simulink model "sampleModel52"  (R2021b)
settings: Solver=VariableStepAuto  StartTime=0.0  StopTime=10.0  RelTol=1e-3
undefined symbols (not defined in the file or in its folder): magnitude
libraries: simulink x3
settings Model: Creator=user  LastModifiedBy=user

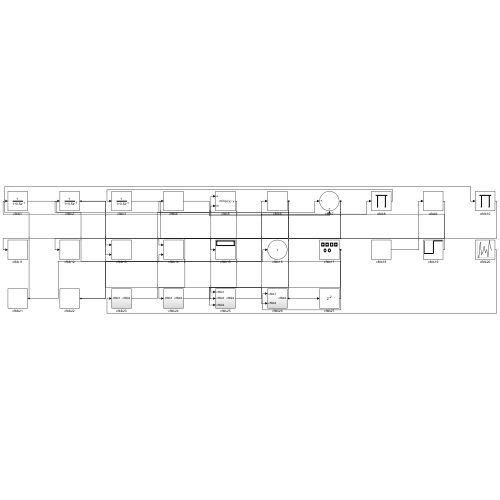
[thumbnail: Simulink's stored preview of the top-level diagram]
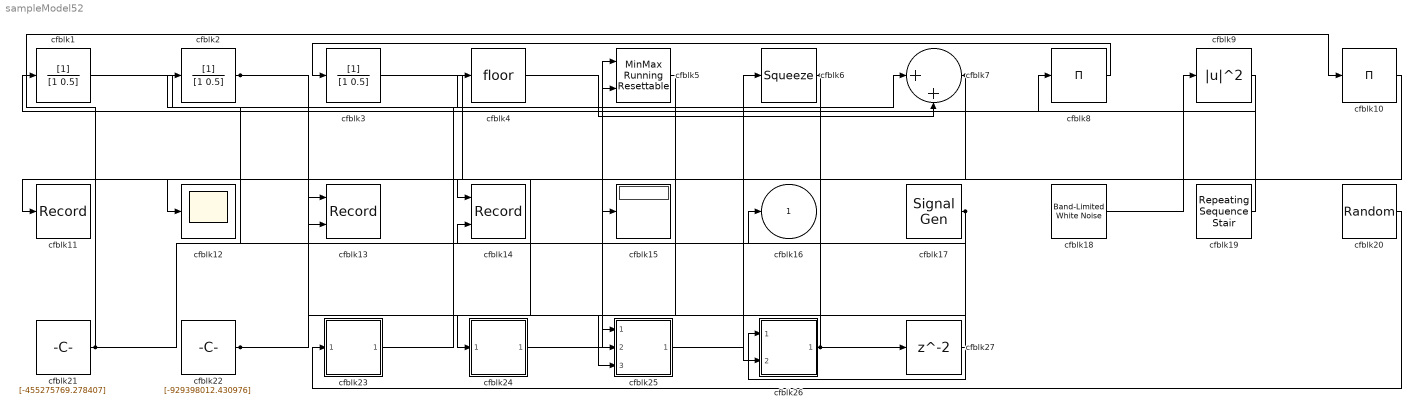
== system sampleModel52 ==
  cfblk1 : DiscreteFilter  SampleTime=1
  cfblk10 : Product  Inputs=*
  cfblk11 : Record  FileSettingsInternal="{\"entries\":[{\"content\":{\"excelSettings\":{\"content\":{},\"type\":\"Streamout.ExcelSettings\"}},\"type\":\"Streamout.FileSettingStorage\",\"uuid\":\"a58b4b1c-998b-4355-a435-f907c9f0cfa4\"}],\"packageUris\":[\"http://schema.mathworks.com/mf0/streamout_blocks/R2020a\"],\"version\":\"1.0\"}"  SignalsInternal="{\"entries\":[{\"content\":{\"signals\":[{\"content\":{\"blockPath\":[\"sampleModel52/cfblk11\"],\"channel\":[],\"dimensions\":[1],\"domain\":\"sampleModel52/cfblk11\",\"lineColor\":\"#7e2f8e\",\"plots\":[1],\"port\":1,\"sid\":[\"\"],\"signalID\":1924,\"signalName\":\"cfblk7\"},\"type\":\"RecordBlkView.Signal\",\"uuid\":\"1dc196f0-91c3-475e-b789-84529fa057b9\"}]},\"type\":\"RecordBlkView.InputSignals\",\"uuid\":\"2605bb36-49aa-42f8-ae4a-f3c9d7892acb\"}],\"packageUris\":[\"http://schema.mathworks.com/mf0/streamout_blocks/R2020a\"],\"version\":\"1.0\"}"  VisualizationBindings="{\"sparklinesplugin\":{\"info\":[{\"bindingParametersList\":[],\"subplotID\":1}]}}"
  cfblk12 : Scope
  cfblk13 : Record  FileSettingsInternal="{\"entries\":[{\"content\":{\"excelSettings\":{\"content\":{},\"type\":\"Streamout.ExcelSettings\"}},\"type\":\"Streamout.FileSettingStorage\",\"uuid\":\"a853c141-9c48-4e83-8f9d-dc3868db9c3d\"}],\"packageUris\":[\"http://schema.mathworks.com/mf0/streamout_blocks/R2020a\"],\"version\":\"1.0\"}"  Layout=[1 1]  SignalsInternal="{\"entries\":[{\"content\":{\"signals\":[{\"content\":{\"blockPath\":[\"sampleModel52/cfblk13\"],\"channel\":[],\"dimensions\":[1],\"domain\":\"sampleModel52/cfblk13\",\"lineColor\":\"#a2142f\",\"plots\":[1],\"port\":1,\"sid\":[\"\"],\"signalID\":1928,\"signalName\":\"cfblk2\"},\"type\":\"RecordBlkView.Signal\",\"uuid\":\"908df438-15f8-4bc3-abdb-438375b4e37a\"},{\"content\":{\"blockPath\":[\"sampleModel52/cfblk13\"],\"channel\":[],\"dimensions\":[1],\"domain\":\"sampleModel52/cfblk13\",\"lineColor\":\"#139fff\",\"plots\":[1],\"port\":2,\"sid\":[\"\"],\"signalID\":1932,\"signalName\":\"cfblk6\"},\"type\":\"RecordBlkView.Signal\",\"uuid\":\"b8a15044-644c-4ec7-b516-ee21329c45a6\"}]},\"type\":\"RecordBlkView.InputSignals\",\"uuid\":\"c864b28a-6f49-4c15-b914-3490e80f919b\"}],\"packageUris\":[\"http://schema.mathworks.com/mf0/streamout_blocks/R2020a\"],\"version\":\"1.0\"}"  VisualizationBindings="{\"xyplotplugin\":{\"info\":[{\"series\":[{\"bindingParametersList\":[{\"parameter\":\"X-Axis\",\"signalID\":1928,\"signalName\":\"cfblk2\"},{\"parameter\":\"Y-Axis\",\"signalID\":1932,\"signalName\":\"cfblk6\"}],\"seriesID\":31757}],\"subplotID\":1}]}}"  CompatibilityTag=XY
  cfblk14 : Record  FileSettingsInternal="{\"entries\":[{\"content\":{\"excelSettings\":{\"content\":{},\"type\":\"Streamout.ExcelSettings\"}},\"type\":\"Streamout.FileSettingStorage\",\"uuid\":\"8f974883-58d1-4d46-9776-bf738691c03f\"}],\"packageUris\":[\"http://schema.mathworks.com/mf0/streamout_blocks/R2020a\"],\"version\":\"1.0\"}"  Layout=[1 1]  SignalsInternal="{\"entries\":[{\"content\":{\"signals\":[{\"content\":{\"blockPath\":[\"sampleModel52/cfblk14\"],\"channel\":[],\"dimensions\":[1],\"domain\":\"sampleModel52/cfblk14\",\"lineColor\":\"#a2142f\",\"plots\":[1],\"port\":1,\"sid\":[\"\"],\"signalID\":1936,\"signalName\":\"cfblk10\"},\"type\":\"RecordBlkView.Signal\",\"uuid\":\"575c55aa-4651-47c4-ad9b-60ba5c6a26c1\"},{\"content\":{\"blockPath\":[\"sampleModel52/cfblk14\"],\"channel\":[],\"dimensions\":[1],\"domain\":\"sampleModel52/cfblk14\",\"lineColor\":\"#139fff\",\"plots\":[1],\"port\":2,\"sid\":[\"\"],\"signalID\":1940,\"signalName\":\"cfblk22\"},\"type\":\"RecordBlkView.Signal\",\"uuid\":\"c771c011-64f7-4db3-b786-dbe9e206db49\"}]},\"type\":\"RecordBlkView.InputSignals\",\"uuid\":\"50dc96e0-5e9f-484c-b19f-096910dc600a\"}],\"packageUris\":[\"http://schema.mathworks.com/mf0/streamout_blocks/R2020a\"],\"version\":\"1.0\"}"  VisualizationBindings="{\"xyplotplugin\":{\"info\":[{\"series\":[{\"bindingParametersList\":[{\"parameter\":\"X-Axis\",\"signalID\":1936,\"signalName\":\"cfblk10\"},{\"parameter\":\"Y-Axis\",\"signalID\":1940,\"signalName\":\"cfblk22\"}],\"seriesID\":45420}],\"subplotID\":1}]}}"  CompatibilityTag=XY
  cfblk15 : Display
  cfblk17 : SignalGenerator  Amplitude=[128217148.273613]
  cfblk18 : simulink/Sources/Band-Limited White Noise  Cov=[3167072841.579786]  Ts=0.1  seed=[7049518769.000000]
  cfblk19 : simulink/Sources/Repeating Sequence Stair  OutValues=[-856462666.606302, -817931228.533560]  tsamp=-1  OutMin=[]  OutMax=[]  OutDataTypeStr=double  OutputDataTypeScalingMode=double  OutDataType=fixdt(0,8)  ConRadixGroup=Best Precision: Vector-wise  OutScaling=2^-12
  cfblk2 : DiscreteFilter  SampleTime=1
  cfblk20 : UniformRandomNumber  Minimum=[-8152621950.425169]  Maximum=[1925676936.090019]  Seed=[15647308.000000]  SampleTime=0.1
  cfblk21 : Constant  Value=[-455275769.278407]  SampleTime=1
  cfblk22 : Constant  Value=[-929398012.430976]  SampleTime=1
  cfblk23 : Subsystem
  cfblk24 : Subsystem
  cfblk25 : Subsystem
  cfblk26 : Subsystem
  cfblk27 : Delay  SampleTime=1
  cfblk3 : DiscreteFilter  SampleTime=1
  cfblk4 : Rounding
  cfblk5 : simulink/Math Operations/MinMax Running Resettable  Function=min  vinit=0.0
  cfblk6 : Squeeze
  cfblk7 : Sum  Inputs=|++
  cfblk8 : Product  Inputs=*
  cfblk9 : Math  Operator=magnitude^2  SaturateOnIntegerOverflow=on
  cfblk16 : Outport
  wires:
  cfblk10/1 -> cfblk14/1
  cfblk8/1 -> cfblk3/1
  cfblk1/1 -> cfblk7/1
  cfblk24/1(cfblk2) -> cfblk5/1
  cfblk3/1 -> cfblk15/1
  cfblk26/1(cfblk2) -> cfblk4/1, cfblk27/1
  cfblk7/1 -> cfblk24/1(cfblk1), cfblk11/1
  cfblk21/1 -> cfblk10/1, cfblk6/1
  cfblk18/1 -> cfblk9/1
  cfblk17/1 -> cfblk26/1(cfblk1), cfblk25/3(cfblk4)
  cfblk20/1 -> cfblk23/1(cfblk1)
  cfblk23/1(cfblk2) -> cfblk5/2
  cfblk19/1 -> cfblk1/1
  cfblk5/1 -> cfblk12/1
  cfblk22/1 -> cfblk16/1, cfblk14/2
  cfblk25/1(cfblk2) -> cfblk8/1
  cfblk9/1 -> cfblk25/1(cfblk1)
  cfblk2/1 -> cfblk13/1, cfblk26/2(cfblk4)
  cfblk6/1 -> cfblk13/2, cfblk25/2(cfblk3)
  cfblk4/1 -> cfblk7/2
  cfblk27/1 -> cfblk2/1

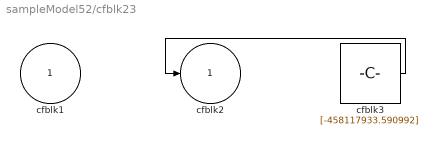
== system sampleModel52/cfblk23 ==
  cfblk1 : Inport
  cfblk3 : Constant  Value=[-458117933.590992]  SampleTime=1
  cfblk2 : Outport
  wires:
  cfblk3/1 -> cfblk2/1

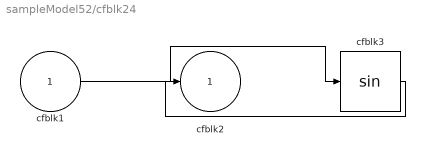
== system sampleModel52/cfblk24 ==
  cfblk1 : Inport
  cfblk3 : Trigonometry
  cfblk2 : Outport
  wires:
  cfblk1/1 -> cfblk3/1
  cfblk3/1 -> cfblk2/1

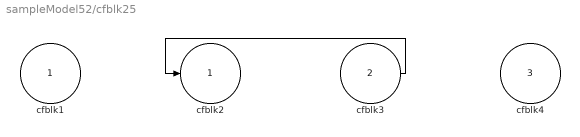
== system sampleModel52/cfblk25 ==
  cfblk1 : Inport
  cfblk3 : Inport  Port=2
  cfblk4 : Inport  Port=3
  cfblk2 : Outport
  wires:
  cfblk3/1 -> cfblk2/1

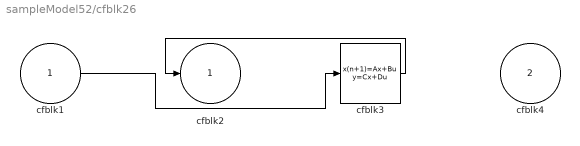
== system sampleModel52/cfblk26 ==
  cfblk1 : Inport
  cfblk4 : Inport  Port=2
  cfblk3 : DiscreteStateSpace
  cfblk2 : Outport
  wires:
  cfblk3/1 -> cfblk2/1
  cfblk1/1 -> cfblk3/1
